simulink model "blobDetect_RP_2"  (R2013b)
settings: Solver=FixedStepDiscrete  StartTime=0.0  StopTime=inf  RelTol=1e-3
PreLoadFcn:
  | load projectionMatrix.mat
undefined symbols (not defined in the file or in its folder): delay
libraries: visionstatistics x3, dspbuff3 x2, embdlinuxlib x2, dspindex x2, visiontextngfix x1, visionanalysis x1
settings Model: SimulationMode=external  ExtModeTrigDuration=100  Creator=vleung  LastModifiedBy=vleung
settings OptimizationCC: OptimizeModelRefInitCode=on  LifeSpan=1
settings DebuggingCC: SolverPrmCheckMsg=none
settings HardwareCC: ProdLargestAtomicInteger=Long  ProdLargestAtomicFloat=Double  ProdEndianess=LittleEndian  ProdHWDeviceType=ARM Compatible->ARM Cortex
settings RTWCC: SystemTargetFile=realtime.tlc  GenerateMakefile=off  TemplateMakefile=realtime.tmf  Description=Run on Target Hardware  RTWVerbose=off  ProcessScript=realtime_make_rtw_hook
settings STFCustomTargetCC: TargetLibSuffix=.a  GenerateSampleERTMain=on  ERTCustomFileBanners=on  SupportNonInlinedSFcns=off  SupportVariableSizeSignals=on  MATLABClassNameForMDSCustomization=Simulink.SoftwareTarget.ERTCustomization  GRTInterface=off  SystemTargetFile=realtime.tlc
settings ERTTargetCC: CodeReplacementLibrary=ANSI_C  GenerateSampleERTMain=on  ParMdlRefBuildCompliant=off  CompOptLevelCompliant=off  ConcurrentExecutionCompliant=off  CombineOutputUpdateFcns=off  ERTFirstTimeCompliant=off  SupportContinuousTime=on  SupportVariableSizeSignals=on  ModelStepFunctionPrototypeControlCompliant=off  CPPClassGenCompliant=off  ExtModeMexArgs='10.10.10.10' 0 17725  InlinedParameterPlacement=NonHierarchical  ERTSrcFileBannerTemplate=realtime_code_template.cgt  ERTHdrFileBannerTemplate=realtime_code_template.cgt  ERTDataSrcFileTemplate=realtime_code_template.cgt  ERTDataHdrFileTemplate=realtime_code_template.cgt  ERTCustomFileTemplate=realtime_file_process.tlc

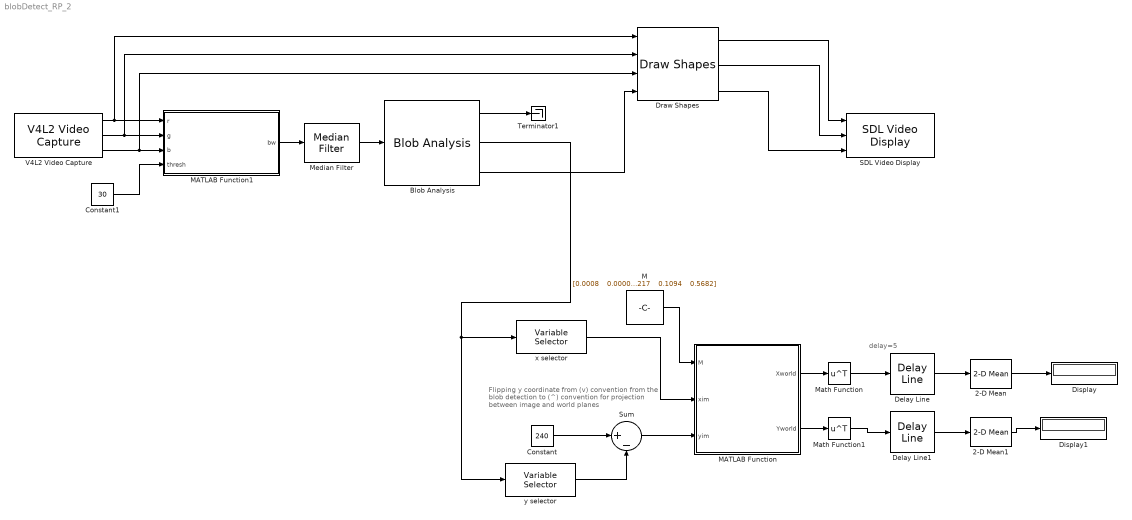
== system blobDetect_RP_2 ==
  note: delay=5
  note: Flipping y coordinate from (v) convention from
      | the blob detection to (^) convention for projection
      | between image and world planes
  2-D Mean : visionstatistics/2-D Mean  run=off  reset_popup=None  directionMode=Each column  dimension=1  treatSBRowAsCol=on  roiEnable=off  roiType=Rectangles  roiPortion=Entire ROI  roiOutput=Individual statistics for each ROI  roiFlag=off  outputDataTypeStr=Inherit: Same as accumulator  outputLastDataTypeStr=Inherit: Same as accumulator  outputMin=[]  outputMax=[]  accumMode=Binary point scaling  accumWordLength=32  accumFracLength=0  accumDataTypeStr=fixdt([],32,0)  accumLastDataTypeStr=fixdt([],32,0)  roundingMode=Floor  overflowMode=off
  2-D Mean1 : visionstatistics/2-D Mean  run=off  reset_popup=None  directionMode=Each column  dimension=1  treatSBRowAsCol=on  roiEnable=off  roiType=Rectangles  roiPortion=Entire ROI  roiOutput=Individual statistics for each ROI  roiFlag=off  outputDataTypeStr=Inherit: Same as accumulator  outputLastDataTypeStr=Inherit: Same as accumulator  outputMin=[]  outputMax=[]  accumMode=Binary point scaling  accumWordLength=32  accumFracLength=0  accumDataTypeStr=fixdt([],32,0)  accumLastDataTypeStr=fixdt([],32,0)  roundingMode=Floor  overflowMode=off
  Blob Analysis : visionstatistics/Blob Analysis  Tag=vipblks_row_conv  area=on  centroid=on  bBox=on  majorAxis=off  minorAxis=off  angle=off  eccentricity=off  equivDiameterSq=off  extent=off  perimeter=off  maxBlobs=6  warnIfNumBlobsExceeded=off  isCount=off  useMinArea=on  minArea=50  useMaxArea=off  maxArea=intmax('uint32')  excludeBorderBlob=on  outDT=single  isOutVarDim=off  isFill=on  fillValues=-1  conn=8  isLabel=off  outputMode=Binary point scaling  outputWordLength=32  outputFracLength=16  firstCoeffMode=Binary point scaling  firstCoeffWordLength=16  firstCoeffFracLength=14  secondCoeffMode=Binary point scaling  secondCoeffWordLength=32  secondCoeffFracLength=16  accumMode=Binary point scaling  accumWordLength=32  accumFracLength=0  prodOutputMode=Binary point scaling  prodOutputWordLength=32  prodOutputFracLength=16  roundingMode=Floor  overflowMode=off
  Constant : Constant  Value=240  OutDataTypeStr=single
  Constant1 : Constant  Value=30  OutDataTypeStr=single
  Delay Line : dspbuff3/Delay Line  siz=6*delay  ic=0  directfeed=off  enable_output=off  hold_output=off  TreatMby1Signals=One channel
  Delay Line1 : dspbuff3/Delay Line  siz=6*delay  ic=0  directfeed=off  enable_output=off  hold_output=off  TreatMby1Signals=One channel
  Display : Display
  Display1 : Display
  Draw Shapes : visiontextngfix/Draw Shapes  shape=Rectangles  fill=off  fillClrSource=Specify via dialog  display=User-specified value  intensity=200  color=[0 0 0]  opacity=0.6  viewport=Entire image  antialiasing=off  inType=Obsolete  imagePorts=Separate color signals  prodOutputMode=Binary point scaling  prodOutputWordLength=32  prodOutputFracLength=14  memoryMode=Specify word length  memoryWordLength=16  memoryFracLength=15  roundingMode=Floor  overflowMode=off
  M : Constant  Value="[0.0008    0.0000   -0.0000; 0.0000    0.0004   -0.0016; -0.1217    0.1094    0.5682]"  VectorParams1D=off  OutDataTypeStr=single
  MATLAB Function : MATLAB Function  TreatAsAtomicUnit=on
  MATLAB Function1 : MATLAB Function  TreatAsAtomicUnit=on
  Math Function : Math  Operator=transpose  SaturateOnIntegerOverflow=on
  Math Function1 : Math  Operator=transpose  SaturateOnIntegerOverflow=on
  Median Filter : visionanalysis/Median Filter  nghbood=[3 3]  outSize=Same as input port I  padType=Constant  padSrc=Specify via dialog  padVal=0  roundingMode=Floor  overflowMode=off
  SDL Video Display : embdlinuxlib/SDL Video Display  pixelFormat=RGB  pixelOrder=Planar  rowMajor=on  blockPlatform=Raspberry Pi
  Sum : Sum  Inputs=|+-
  Terminator1 : Terminator
  V4L2 Video Capture : embdlinuxlib/V4L2 Video Capture  m_devName='/dev/video0'  roi=[0, 0, 640, 480]  imSizeSelection=320x240  imSize=[640, 480]  pixelFormat=RGB  pixelOrder=Planar  sampleTime=1/10  simOutput=Colorbars  blockPlatform=Raspberry Pi
  x selector : dspindex/Variable Selector  NumInputs=1  rowsOrCols=Columns  IdxMode=Fixed  Elements=1  ZerOneIdxMode=One-based  errmode=Generate Error  FillMode=on  FillValues=0
  y selector : dspindex/Variable Selector  NumInputs=1  rowsOrCols=Columns  IdxMode=Fixed  Elements=2  ZerOneIdxMode=One-based  errmode=Generate Error  FillMode=on  FillValues=0
  wires:
  Blob Analysis/2 -> y selector/1, x selector/1
  y selector/1 -> Sum/2
  Constant/1 -> Sum/1
  Sum/1 -> MATLAB Function/3(yim)
  x selector/1 -> MATLAB Function/2(xim)
  MATLAB Function/1(Xworld) -> Math Function/1
  MATLAB Function/2(Yworld) -> Math Function1/1
  M/1 -> MATLAB Function/1(M)
  Delay Line/1 -> 2-D Mean/1
  2-D Mean/1 -> Display/1
  Math Function/1 -> Delay Line/1
  Math Function1/1 -> Delay Line1/1
  Delay Line1/1 -> 2-D Mean1/1
  2-D Mean1/1 -> Display1/1
  V4L2 Video Capture/3 -> Draw Shapes/3, MATLAB Function1/3(b)
  V4L2 Video Capture/2 -> Draw Shapes/2, MATLAB Function1/2(g)
  V4L2 Video Capture/1 -> Draw Shapes/1, MATLAB Function1/1(r)
  Draw Shapes/3 -> SDL Video Display/3
  Draw Shapes/1 -> SDL Video Display/1
  Draw Shapes/2 -> SDL Video Display/2
  Constant1/1 -> MATLAB Function1/4(thresh)
  Median Filter/1 -> Blob Analysis/1
  Blob Analysis/3 -> Draw Shapes/4
  Blob Analysis/1 -> Terminator1/1
  MATLAB Function1/1(bw) -> Median Filter/1

== matlab function blobDetect_RP_2/MATLAB Function1 ==
  data: r input; bw output; g input; b input; thresh input
function bw = greenDetect(r, g, b, thresh)
%#codegen

justGreen = single(g) - single(r)/2 - single(b)/2;

bw = justGreen > thresh;

== matlab function blobDetect_RP_2/MATLAB Function ==
  data: M input; Xworld output; xim input; yim input; Yworld output
function [Xworld, Yworld] = image2world(M, xim, yim)
%#codegen

% Inputs: xim = [nx1] vector of x-coordinate in image plane
%         yim = [nx1] vector of y-coordinate in image plane
%         
%         For the image coordinates, origin is bottom left, convention:
%         x (>), y(^)
%
% Outputs: Xworld = [nx1] vector of x-coordinates in world plane
%          Yworld = [nx1] vector of y-coordinates in world plane
%          
%          For the world coordinates, robot at (X,Y) = (0,0)
%

% if size(xim, 2) > size(xim, 1)
%     xim = xim' ;
% end
% 
% if size(yim, 2) > size(yim, 1)
%     yim = yim' ;
% end
    
% [Xworld,Yworld] = transformPointsInverse(t_world2im, xim, yim) ;
% transformPointsInverse does not support codegen, but can get code from
% its class projective2d.

% M = inv( t_world2im );
u = M(1,1).*xim + M(2,1).*yim + M(3,1);
v = M(1,2).*xim + M(2,2).*yim + M(3,2);
w = M(1,3).*xim + M(2,3).*yim + M(3,3);

Xworld = u./w ;
Yworld = v./w ;

% limite the minimum Yworld to 0
Yworld = max([Yworld, zeros(size(Yworld))],[],2) ;
